simulink model "aterragem_ILS_GulfVsim"  (R2019b)
settings: Solver=VariableStepAuto  StartTime=0.0  StopTime=300  RelTol=1e-3
values from neighbouring files (symbols this model uses):
  aa0 = 7.17*deg    (= 0.125140107368)    [variaveis_GulfV.m]
  ah = [ ... (first row only)    [aterragem_ILS_GulfV.m]
  bh = [ ... (first row only)    [aterragem_ILS_GulfV.m]
  Fh = inv(Gh)    [aterragem_ILS_GulfV.m]
  h0 = 500    [variaveis_GulfV.m]
  kh_lqr = lqr(ah,bh,qh,rh)    [aterragem_ILS_GulfV.m]
  tt0 = gg0+aa0    (= 0.125140107368)    [variaveis_GulfV.m]
  u0 = 105.1*kn    (= 54.06344)    [variaveis_GulfV.m]
libraries: simulink x4
settings Model: Creator=Admin  LastModifiedBy=PedroNeves

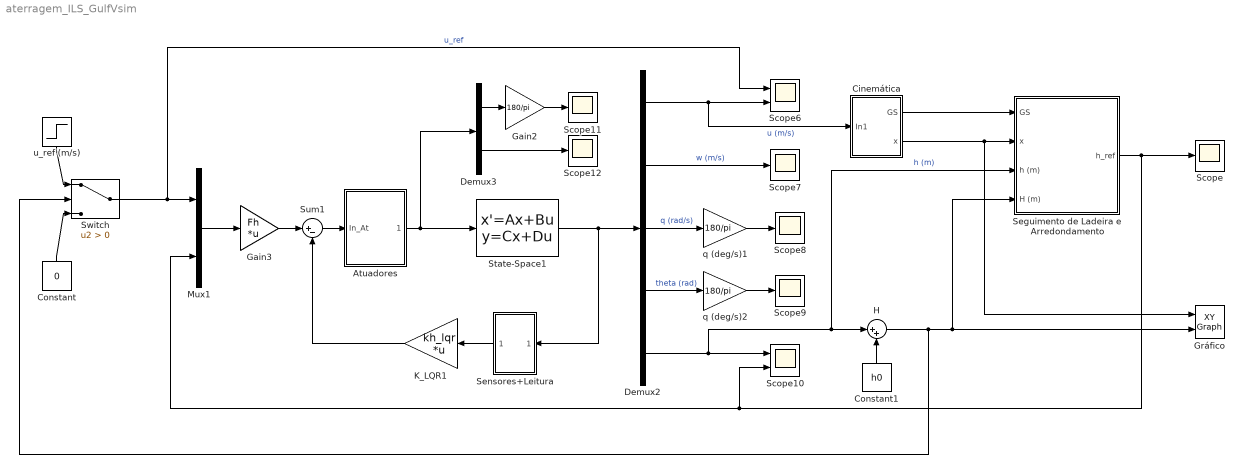
== system aterragem_ILS_GulfVsim ==
  Atuadores : Subsystem
  Cinemática : Subsystem
  Constant : Constant  Value=0
  Constant1 : Constant  Value=h0
  Demux2 : Demux  Outputs=5
  Demux3 : Demux  Outputs=2
  Gain2 : Gain  Gain=180/pi
  Gain3 : Gain  Gain=Fh  Multiplication=Matrix(K*u)
  Gráfico : simulink/Sinks/XY Graph  xmin=-10000  xmax=20000  ymin=-7  ymax=600  st=-1
  H : Sum  Inputs=|++
  K_LQR1 : Gain  Gain=kh_lqr  Multiplication=Matrix(K*u)
  Mux1 : Mux  Inputs=2
  Scope{,7..9,11..12} (6 alike) : Scope
  Scope10 : Scope  NumInputPorts=2
  Scope6 : Scope  NumInputPorts=2
  Seguimento de Ladeira e Arredondamento : Subsystem
  Sensores+Leitura : Subsystem
  State-Space1 : StateSpace  A=ah  B=bh  C=eye(5)  D=zeros(5,2)  InitialCondition=0
  Sum1 : Sum  Inputs=|+-
  Switch : Switch  Criteria=u2 > Threshold
  q (deg/s)1 : Gain  Gain=180/pi
  q (deg/s)2 : Gain  Gain=180/pi
  u_ref (m/s) : Step  SampleTime=0
  wires:
  Demux2/1 -> Cinemática/1(In1), Scope6/2  "u (m/s)"
  Demux2/2 -> Scope7/1  "w (m/s)"
  Demux2/5 -> H/1, Seguimento de Ladeira e Arredondamento/3(h (m)), Scope10/1  "h (m)"
  State-Space1/1 -> Sensores+Leitura/1(In1), Demux2/1
  Demux2/3 -> q (deg/s)1/1  "q (rad/s)"
  q (deg/s)1/1 -> Scope8/1
  q (deg/s)2/1 -> Scope9/1
  Demux2/4 -> q (deg/s)2/1  "theta (rad)"
  Gain2/1 -> Scope11/1
  Demux3/1 -> Gain2/1
  Demux3/2 -> Scope12/1
  K_LQR1/1 -> Sum1/2
  Gain3/1 -> Sum1/1
  Seguimento de Ladeira e Arredondamento/1(h_ref) -> Mux1/2, Scope10/2, Scope/1
  Mux1/1 -> Gain3/1
  Cinemática/1(GS) -> Seguimento de Ladeira e Arredondamento/1(GS)
  Cinemática/2(x) -> Gráfico/1, Seguimento de Ladeira e Arredondamento/2(x)
  H/1 -> Switch/2, Seguimento de Ladeira e Arredondamento/4(H (m)), Gráfico/2
  Constant1/1 -> H/2
  u_ref (m/s)/1 -> Switch/1
  Switch/1 -> Scope6/1, Mux1/1  "u_ref"
  Constant/1 -> Switch/3
  Sum1/1 -> Atuadores/1(In_At)
  Atuadores/1(Out_At) -> Demux3/1, State-Space1/1
  Sensores+Leitura/1(Out2) -> K_LQR1/1

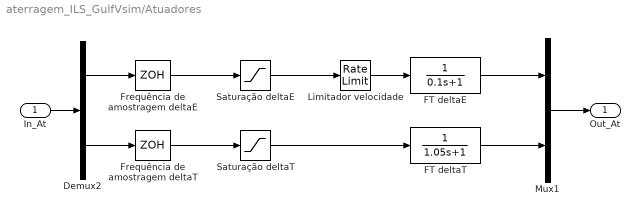
== system aterragem_ILS_GulfVsim/Atuadores ==
  In_At : Inport
  Demux2 : Demux  Outputs=2
  FT deltaE : TransferFcn  Denominator=[0.1 1]
  FT deltaT : TransferFcn  Denominator=[1.05 1]
  Frequência de amostragem deltaT : ZeroOrderHold  SampleTime=-1
  "Frequência de amostragem deltaE " : ZeroOrderHold  SampleTime=1/40
  Limitador velocidade : RateLimiter  SampleTimeMode=inherited
  Mux1 : Mux  Inputs=2
  Saturação deltaE : Saturate  UpperLimit=28*(pi/180)  LowerLimit=-21*(pi/180)
  Saturação deltaT : Saturate  UpperLimit=0.27  LowerLimit=-0.73
  Out_At : Outport
  wires:
  Demux2/2 -> Frequência de amostragem deltaT/1
  "Frequência de amostragem deltaE "/1 -> Saturação deltaE/1
  Demux2/1 -> "Frequência de amostragem deltaE "/1
  Mux1/1 -> Out_At/1
  FT deltaE/1 -> Mux1/1
  In_At/1 -> Demux2/1
  Saturação deltaE/1 -> Limitador velocidade/1
  Saturação deltaT/1 -> FT deltaT/1
  Limitador velocidade/1 -> FT deltaE/1
  Frequência de amostragem deltaT/1 -> Saturação deltaT/1
  FT deltaT/1 -> Mux1/2

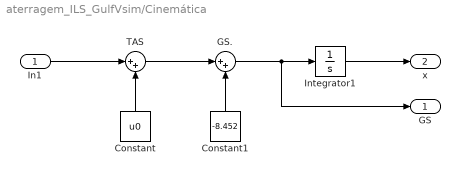
== system aterragem_ILS_GulfVsim/Cinemática ==
  In1 : Inport
  Constant : Constant  Value=u0
  Constant1 : Constant  Value=-8.452
  GS. : Sum  Inputs=|++
  Integrator1 : Integrator
  TAS : Sum  Inputs=|++
  GS : Outport
  x : Outport  Port=2
  wires:
  Constant1/1 -> GS./2
  TAS/1 -> GS./1
  GS./1 -> GS/1, Integrator1/1
  Constant/1 -> TAS/2
  In1/1 -> TAS/1
  Integrator1/1 -> x/1

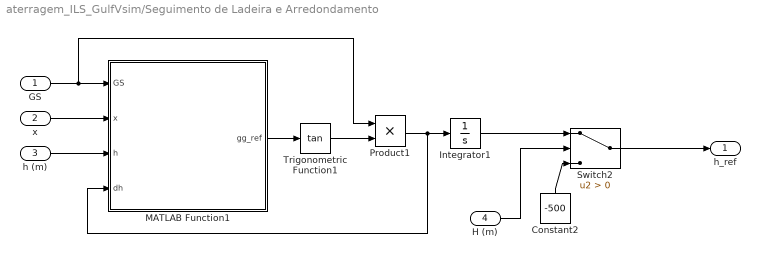
== system aterragem_ILS_GulfVsim/Seguimento de Ladeira e Arredondamento ==
  GS : Inport
  x : Inport  Port=2
  h (m) : Inport  Port=3
  H (m) : Inport  Port=4
  Constant2 : Constant  Value=-500
  Integrator1 : Integrator
  MATLAB Function1 : MATLAB Function  TreatAsAtomicUnit=on
  Product1 : Product
  Switch2 : Switch  Criteria=u2 > Threshold
  Trigonometric Function1 : Trigonometry  Operator=tan
  h_ref : Outport
  wires:
  Trigonometric Function1/1 -> Product1/2
  Product1/1 -> MATLAB Function1/4(dh), Integrator1/1
  Integrator1/1 -> Switch2/1
  GS/1 -> Product1/1, MATLAB Function1/1(GS)
  H (m)/1 -> Switch2/2
  Constant2/1 -> Switch2/3
  x/1 -> MATLAB Function1/2(x)
  MATLAB Function1/1(gg_ref) -> Trigonometric Function1/1
  Switch2/1 -> h_ref/1
  h (m)/1 -> MATLAB Function1/3(h)

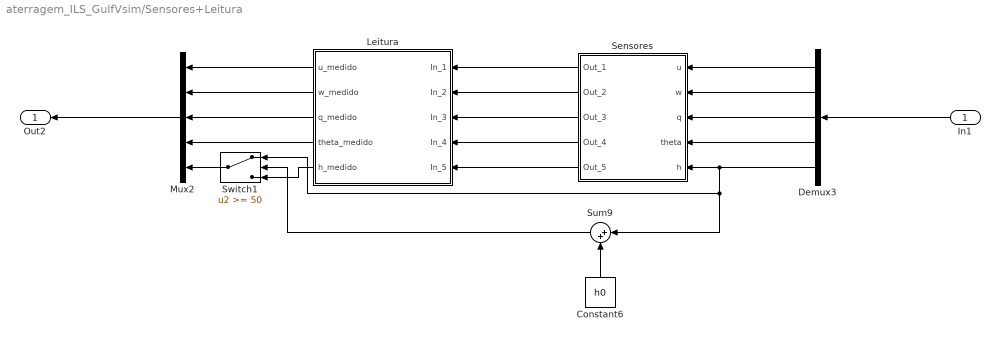
== system aterragem_ILS_GulfVsim/Sensores+Leitura ==
  In1 : Inport
  Constant6 : Constant  Value=h0
  Demux3 : Demux  Outputs=5
  Leitura : Subsystem
  Mux2 : Mux  Inputs=5
  Sensores : Subsystem
  Sum9 : Sum  Inputs=|++
  Switch1 : Switch  Threshold=50
  Out2 : Outport
  wires:
  Mux2/1 -> Out2/1
  In1/1 -> Demux3/1
  Leitura/1(u_medido) -> Mux2/1
  Leitura/2(w_medido) -> Mux2/2
  Leitura/3(q_medido) -> Mux2/3
  Demux3/1 -> Sensores/1(u)
  Demux3/2 -> Sensores/2(w)
  Demux3/3 -> Sensores/3(q)
  Sensores/1(Out_1) -> Leitura/1(In_1)
  Sensores/2(Out_2) -> Leitura/2(In_2)
  Sensores/3(Out_3) -> Leitura/3(In_3)
  Sensores/4(Out_4) -> Leitura/4(In_4)
  Demux3/4 -> Sensores/4(theta)
  Demux3/5 -> Sum9/1, Switch1/1, Sensores/5(h)
  Leitura/4(theta_medido) -> Mux2/4
  Sensores/5(Out_5) -> Leitura/5(In_5)
  Switch1/1 -> Mux2/5
  Leitura/5(h_medido) -> Switch1/3
  Sum9/1 -> Switch1/2
  Constant6/1 -> Sum9/2

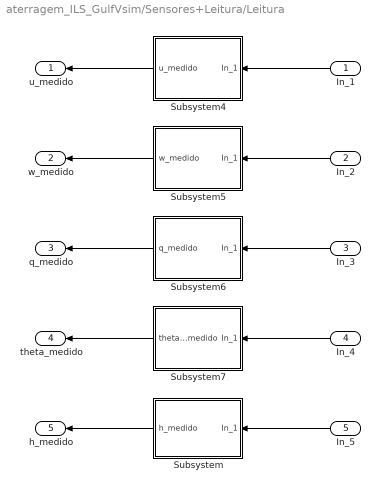
== system aterragem_ILS_GulfVsim/Sensores+Leitura/Leitura ==
  In_1 : Inport
  In_2 : Inport  Port=2
  In_3 : Inport  Port=3
  In_4 : Inport  Port=4
  In_5 : Inport  Port=5
  Subsystem : Subsystem
  Subsystem4 : Subsystem
  Subsystem5 : Subsystem
  Subsystem6 : Subsystem
  Subsystem7 : Subsystem
  u_medido : Outport
  w_medido : Outport  Port=2
  q_medido : Outport  Port=3
  theta_medido : Outport  Port=4
  h_medido : Outport  Port=5
  wires:
  In_2/1 -> Subsystem5/1(In_1)
  In_4/1 -> Subsystem7/1(In_1)
  Subsystem7/1(theta_medido) -> theta_medido/1
  Subsystem6/1(q_medido) -> q_medido/1
  Subsystem5/1(w_medido) -> w_medido/1
  In_1/1 -> Subsystem4/1(In_1)
  Subsystem4/1(u_medido) -> u_medido/1
  In_3/1 -> Subsystem6/1(In_1)
  In_5/1 -> Subsystem/1(In_1)
  Subsystem/1(h_medido) -> h_medido/1

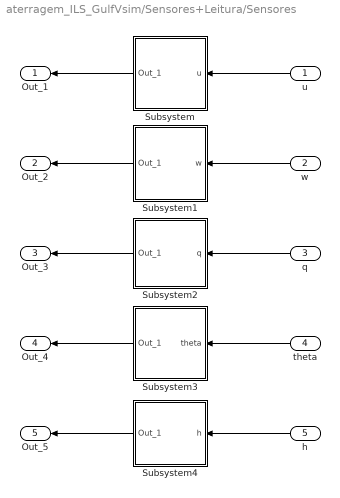
== system aterragem_ILS_GulfVsim/Sensores+Leitura/Sensores ==
  u : Inport
  w : Inport  Port=2
  q : Inport  Port=3
  theta : Inport  Port=4
  h : Inport  Port=5
  Subsystem : Subsystem
  Subsystem1 : Subsystem
  Subsystem2 : Subsystem
  Subsystem3 : Subsystem
  Subsystem4 : Subsystem
  Out_1 : Outport
  Out_2 : Outport  Port=2
  Out_3 : Outport  Port=3
  Out_4 : Outport  Port=4
  Out_5 : Outport  Port=5
  wires:
  Subsystem2/1(Out_1) -> Out_3/1
  q/1 -> Subsystem2/1(q)
  theta/1 -> Subsystem3/1(theta)
  Subsystem3/1(Out_1) -> Out_4/1
  u/1 -> Subsystem/1(u)
  w/1 -> Subsystem1/1(w)
  Subsystem/1(Out_1) -> Out_1/1
  Subsystem1/1(Out_1) -> Out_2/1
  h/1 -> Subsystem4/1(h)
  Subsystem4/1(Out_1) -> Out_5/1

== system aterragem_ILS_GulfVsim/Sensores+Leitura/Leitura/Subsystem ==
  In_1 : Inport
  Constant : Constant  Value=h0
  Gain : Gain  Gain=100
  Gain1 : Gain  Gain=0.3048
  Sum1 : Sum  Inputs=|+-
  h_medido : Outport
  wires:
  Sum1/1 -> h_medido/1
  Gain1/1 -> Sum1/1
  Gain/1 -> Gain1/1
  Constant/1 -> Sum1/2
  In_1/1 -> Gain/1

== system aterragem_ILS_GulfVsim/Sensores+Leitura/Leitura/Subsystem4 ==
  In_1 : Inport
  Constant4 : Constant  Value=u0
  Gain : Gain  Gain=1/0.028
  Gain8 : Gain  Gain=0.5144
  Sum9 : Sum  Inputs=-+|
  u_medido : Outport
  wires:
  Constant4/1 -> Sum9/1
  In_1/1 -> Gain/1
  Gain8/1 -> Sum9/2
  Gain/1 -> Gain8/1
  Sum9/1 -> u_medido/1

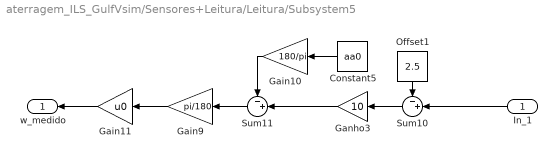
== system aterragem_ILS_GulfVsim/Sensores+Leitura/Leitura/Subsystem5 ==
  In_1 : Inport
  Constant5 : Constant  Value=aa0
  Gain10 : Gain  Gain=180/pi
  Gain11 : Gain  Gain=u0
  Gain9 : Gain  Gain=pi/180
  Ganho3 : Gain  Gain=10
  Offset1 : Constant  Value=2.5
  Sum10 : Sum  Inputs=-+|
  Sum11 : Sum  Inputs=-+|
  w_medido : Outport
  wires:
  Sum11/1 -> Gain9/1
  Constant5/1 -> Gain10/1
  Ganho3/1 -> Sum11/2
  In_1/1 -> Sum10/2
  Gain11/1 -> w_medido/1
  Gain9/1 -> Gain11/1
  Gain10/1 -> Sum11/1
  Offset1/1 -> Sum10/1
  Sum10/1 -> Ganho3/1

== system aterragem_ILS_GulfVsim/Sensores+Leitura/Leitura/Subsystem6 ==
  In_1 : Inport
  Gain12 : Gain  Gain=pi/180
  Ganho4 : Gain  Gain=1/0.06
  q_medido : Outport
  wires:
  Ganho4/1 -> Gain12/1
  In_1/1 -> Ganho4/1
  Gain12/1 -> q_medido/1

== system aterragem_ILS_GulfVsim/Sensores+Leitura/Leitura/Subsystem7 ==
  In_1 : Inport
  Constant6 : Constant  Value=14
  Constant7 : Constant  Value=tt0
  Gain13 : Gain  Gain=pi/180
  Ganho5 : Gain  Gain=30/7
  Sum12 : Sum  Inputs=-+|
  Sum13 : Sum  Inputs=-+|
  theta_medido : Outport
  wires:
  Constant7/1 -> Sum13/1
  Sum12/1 -> Ganho5/1
  Sum13/1 -> theta_medido/1
  Gain13/1 -> Sum13/2
  Ganho5/1 -> Gain13/1
  Constant6/1 -> Sum12/1
  In_1/1 -> Sum12/2

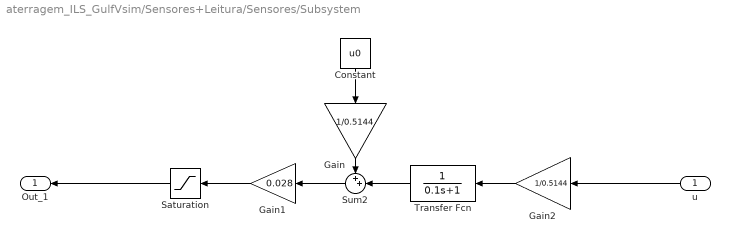
== system aterragem_ILS_GulfVsim/Sensores+Leitura/Sensores/Subsystem ==
  u : Inport
  Constant : Constant  Value=u0
  Gain : Gain  Gain=1/0.5144
  Gain1 : Gain  Gain=0.028
  Gain2 : Gain  Gain=1/0.5144
  Saturation : Saturate  UpperLimit=28  LowerLimit=0
  Sum2 : Sum  Inputs=++|
  Transfer Fcn : TransferFcn  Denominator=[0.1 1]
  Out_1 : Outport
  wires:
  Sum2/1 -> Gain1/1
  Saturation/1 -> Out_1/1
  Gain1/1 -> Saturation/1
  u/1 -> Gain2/1
  Transfer Fcn/1 -> Sum2/2
  Constant/1 -> Gain/1
  Gain2/1 -> Transfer Fcn/1
  Gain/1 -> Sum2/1

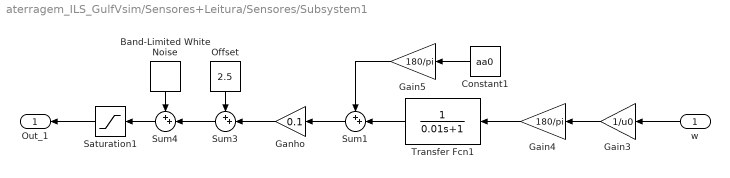
== system aterragem_ILS_GulfVsim/Sensores+Leitura/Sensores/Subsystem1 ==
  w : Inport
  Band-Limited White Noise : simulink/Sources/Band-Limited White Noise  Cov=[(0.005)^2/40]  Ts=1/40  seed=[23341]
  Constant1 : Constant  Value=aa0
  Gain3 : Gain  Gain=1/u0
  Gain4 : Gain  Gain=180/pi
  Gain5 : Gain  Gain=180/pi
  Ganho : Gain  Gain=0.1
  Offset : Constant  Value=2.5
  Saturation1 : Saturate  UpperLimit=5  LowerLimit=0
  Sum1 : Sum  Inputs=++|
  Sum3 : Sum  Inputs=++|
  Sum4 : Sum  Inputs=++|
  Transfer Fcn1 : TransferFcn  Denominator=[0.01 1]
  Out_1 : Outport
  wires:
  Gain5/1 -> Sum1/1
  Sum1/1 -> Ganho/1
  Offset/1 -> Sum3/1
  Constant1/1 -> Gain5/1
  Ganho/1 -> Sum3/2
  Gain4/1 -> Transfer Fcn1/1
  Sum4/1 -> Saturation1/1
  Band-Limited White Noise/1 -> Sum4/1
  Gain3/1 -> Gain4/1
  Transfer Fcn1/1 -> Sum1/2
  Sum3/1 -> Sum4/2
  w/1 -> Gain3/1
  Saturation1/1 -> Out_1/1

== system aterragem_ILS_GulfVsim/Sensores+Leitura/Sensores/Subsystem2 ==
  q : Inport
  Band-Limited White Noise1 : simulink/Sources/Band-Limited White Noise  Cov=[(0.002)^2/40]  Ts=1/40  seed=[23341]
  Gain6 : Gain  Gain=180/pi
  Ganho1 : Gain  Gain=0.06
  Saturation2 : Saturate  UpperLimit=3  LowerLimit=-3
  Sum5 : Sum  Inputs=++|
  Out_1 : Outport
  wires:
  Sum5/1 -> Saturation2/1
  Ganho1/1 -> Sum5/2
  Band-Limited White Noise1/1 -> Sum5/1
  q/1 -> Gain6/1
  Saturation2/1 -> Out_1/1
  Gain6/1 -> Ganho1/1

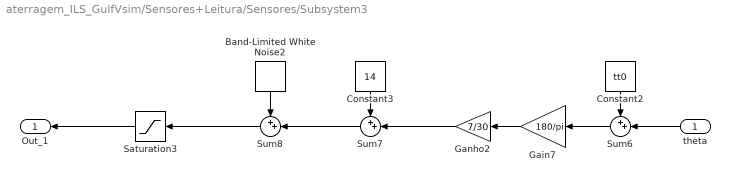
== system aterragem_ILS_GulfVsim/Sensores+Leitura/Sensores/Subsystem3 ==
  theta : Inport
  Band-Limited White Noise2 : simulink/Sources/Band-Limited White Noise  Cov=[((0.25*pi)/180)^2/40]  Ts=1/40  seed=[23341]
  Constant2 : Constant  Value=tt0
  Constant3 : Constant  Value=14
  Gain7 : Gain  Gain=180/pi
  Ganho2 : Gain  Gain=7/30
  Saturation3 : Saturate  UpperLimit=28  LowerLimit=0
  Sum6 : Sum  Inputs=++|
  Sum7 : Sum  Inputs=++|
  Sum8 : Sum  Inputs=++|
  Out_1 : Outport
  wires:
  Sum7/1 -> Sum8/2
  Gain7/1 -> Ganho2/1
  Constant2/1 -> Sum6/1
  Constant3/1 -> Sum7/1
  Sum8/1 -> Saturation3/1
  Ganho2/1 -> Sum7/2
  Sum6/1 -> Gain7/1
  Saturation3/1 -> Out_1/1
  Band-Limited White Noise2/1 -> Sum8/1
  theta/1 -> Sum6/2

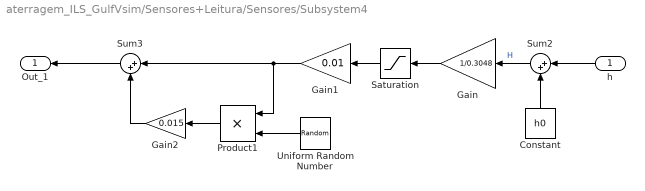
== system aterragem_ILS_GulfVsim/Sensores+Leitura/Sensores/Subsystem4 ==
  h : Inport
  Constant : Constant  Value=h0
  Gain : Gain  Gain=1/0.3048
  Gain1 : Gain  Gain=0.01
  Gain2 : Gain  Gain=0.015
  Product1 : Product
  Saturation : Saturate  UpperLimit=1500  LowerLimit=0
  Sum2 : Sum  Inputs=|++
  Sum3 : Sum  Inputs=|++
  Uniform Random Number : UniformRandomNumber  Minimum=0  SampleTime=0.1
  Out_1 : Outport
  wires:
  Sum2/1 -> Gain/1  "H"
  h/1 -> Sum2/1
  Constant/1 -> Sum2/2
  Product1/1 -> Gain2/1
  Gain2/1 -> Sum3/2
  Gain/1 -> Saturation/1
  Gain1/1 -> Product1/1, Sum3/1
  Saturation/1 -> Gain1/1
  Sum3/1 -> Out_1/1
  Uniform Random Number/1 -> Product1/2

== matlab function aterragem_ILS_GulfVsim/Seguimento de Ladeira e Arredondamento/MATLAB Function1 ==
  data: GS input; x input; h input; dh input; gg_ref output
function gg_ref = fcn(GS, x, h, dh)
deg=pi/180;
ang_ladeira = 3;

x_descida=-450/tan(ang_ladeira*deg);
gg_ref=0;

if(x >= x_descida)
    gg_ref=-ang_ladeira*deg;
end

H = h + 500;

if(H < 50)
   %gg_ref=atan(dh/GS);
    gg_ref = -ang_ladeira*exp(-(50-H)/25)*deg;
    

end

end
